simulink model "saturated_systems_example"  (R2021a)
settings: Solver=VariableStepAuto  StartTime=0.0  StopTime=simTime  RelTol=1e-3
values from neighbouring files (symbols this model uses):
  K_P = 1/abs(freqresp(G_ol,omega_c))    [Anti_windup_example.m]    (also in P_Lead_Lag.m = 1/abs(freqresp(G_ol,omega_c*1i)); Rate_limited_example.m; Rate_limited_exercise.m)
  step_size = 25    [Anti_windup_example.m]    (also in P_Lead_Lag.m = 1)
  tau_i = N_i/omega_c    [Anti_windup_example.m]    (also in P_Lead_Lag.m; Rate_limited_example.m = 0.75; Rate_limited_exercise.m = 0.666666666667)
undefined symbols (not defined in the file or in its folder): den_D, num_D
settings Model: Creator=dimpa  LastModifiedBy=dimpa
settings DataIOCC: Refine=154

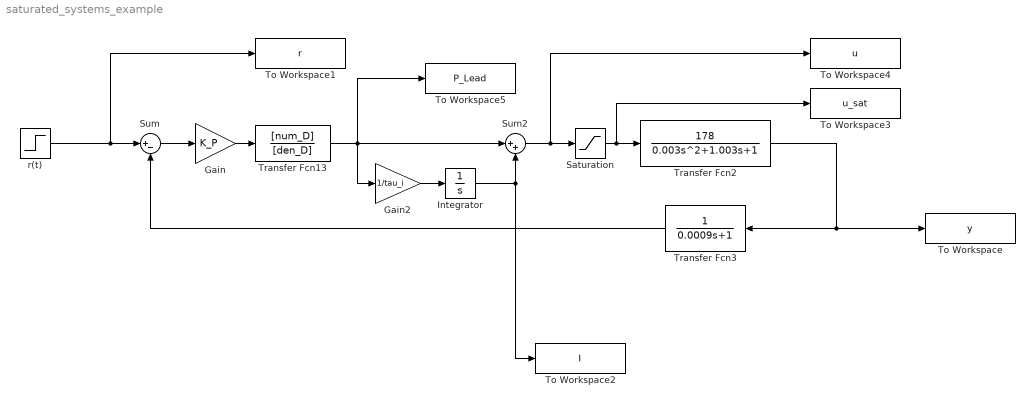
== system saturated_systems_example ==
  Gain : Gain  Gain=K_P
  Gain2 : Gain  Gain=1/tau_i
  Integrator : Integrator
  Saturation : Saturate  UpperLimit=4  LowerLimit=-4
  Sum : Sum  Inputs=|+-
  Sum2 : Sum  Inputs=|++
  To Workspace : ToWorkspace  VariableName=y  SaveFormat=Timeseries  SampleTime=-1
  To Workspace1 : ToWorkspace  VariableName=r  SaveFormat=Timeseries  SampleTime=-1
  To Workspace2 : ToWorkspace  VariableName=I  SaveFormat=Timeseries  SampleTime=-1
  To Workspace3 : ToWorkspace  VariableName=u_sat  SaveFormat=Timeseries  SampleTime=-1
  To Workspace4 : ToWorkspace  VariableName=u  SaveFormat=Timeseries  SampleTime=-1
  To Workspace5 : ToWorkspace  VariableName=P_Lead  SaveFormat=Timeseries  SampleTime=-1
  Transfer Fcn13 : TransferFcn  Numerator=[num_D]  Denominator=[den_D]
  Transfer Fcn2 : TransferFcn  Numerator=[178]  Denominator=[0.003 1.003 1]
  Transfer Fcn3 : TransferFcn  Denominator=[0.0009 1]
  r(t) : Step  Time=0.1  After=step_size  SampleTime=0
  wires:
  Saturation/1 -> To Workspace3/1, Transfer Fcn2/1
  Transfer Fcn2/1 -> To Workspace/1, Transfer Fcn3/1
  r(t)/1 -> To Workspace1/1, Sum/1
  Sum/1 -> Gain/1
  Gain/1 -> Transfer Fcn13/1
  Transfer Fcn3/1 -> Sum/2
  Sum2/1 -> Saturation/1, To Workspace4/1
  Transfer Fcn13/1 -> To Workspace5/1, Gain2/1, Sum2/1
  Gain2/1 -> Integrator/1
  Integrator/1 -> To Workspace2/1, Sum2/2
